simulink library "DQN_Lib (conflicted copy 2023-11-25 155310)"  (R2023b)
settings: Solver=VariableStepAuto  StartTime=0.0  StopTime=10.0  RelTol=1e-3
undefined symbols (not defined in the file): FreqRad, HrmOrd, Init, La, N, R, Ra, TimeStep, Ts, Ts_dqn, Ws
libraries: $bdroot x4, spsMeanVariableFrequencyLib x4, eeTransforms x3, spsabctodq0Lib x2, spsAlphaBetaZerotodq0Lib x1
(part 3 of 8)

== matlab function DQN_Lib (conflicted copy 2023-11-25 155310)/Mult_DQN_Mat ==
  data: X_DQN input; Y_DQN input; Z_DQN output; N parameter; HrmDbl parameter
function Z_DQN   = MultDQN(X_DQN, Y_DQN, N, HrmDbl)

    Xdp = X_DQN(:,1);
    Xdn = X_DQN(:,2);
    Xdz = X_DQN(:,3);
    Xqp = X_DQN(:,4);
    Xqn = X_DQN(:,5);
    Xqz = X_DQN(:,6);
    
    Ydp = Y_DQN(:,1);
    Ydn = Y_DQN(:,2);
    Ydz = Y_DQN(:,3);
    Yqp = Y_DQN(:,4);
    Yqn = Y_DQN(:,5);
    Yqz = Y_DQN(:,6);
    
    Z_DQN = zeros(2*N+1,6);

    Xdc = zeros(6,1);
    Ydc = zeros(6,1);
    Zdc = zeros(6,1);

    Xdc(1) = Xdp(1);
    Xdc(2) = Xdn(1);
    Xdc(3) = Xdz(1);
    Xdc(4) = Xqp(1);
    Xdc(5) = Xqn(1);
    Xdc(6) = Xqz(1);

    Ydc(1) = Ydp(1);
    Ydc(2) = Ydn(1);
    Ydc(3) = Ydz(1);
    Ydc(4) = Yqp(1);
    Ydc(5) = Yqn(1);
    Ydc(6) = Yqz(1);

    a = -0.5+0.866i;
    a2 = -0.5-0.866i;
    T = [1 1 1;1 a a2;1 a2 a];    

    Xdp = [Xdp(2:end); zeros(N-numel(Xdp)+1,1)];
    Ydp = [Ydp(2:end); zeros(N-numel(Ydp)+1,1)];
    Xqp = [Xqp(2:end); zeros(N-numel(Xqp)+1,1)];
    Yqp = [Yqp(2:end); zeros(N-numel(Yqp)+1,1)];
      
    Xdn = [Xdn(2:end); zeros(N-numel(Xdn)+1,1)];
    Ydn = [Ydn(2:end); zeros(N-numel(Ydn)+1,1)];
    Xqn = [Xqn(2:end); zeros(N-numel(Xqn)+1,1)];
    Yqn = [Yqn(2:end); zeros(N-numel(Yqn)+1,1)];
    
    Xdz = [Xdz(2:end); zeros(N-numel(Xdz)+1,1)];
    Ydz = [Ydz(2:end); zeros(N-numel(Ydz)+1,1)];
    Xqz = [Xqz(2:end); zeros(N-numel(Xqz)+1,1)];
    Yqz = [Yqz(2:end); zeros(N-numel(Yqz)+1,1)];
    
    Zdp = zeros(2*N+1,1);
    Zdn = zeros(2*N+1,1);
    Zdz = zeros(2*N+1,1);
    Zqp = zeros(2*N+1,1);
    Zqn = zeros(2*N+1,1);
    Zqz = zeros(2*N+1,1);
    
%    Tad_p =        [0  -0.577350269189626   0.577350269189626;
%    0.666666666666667  -0.333333333333333  -0.333333333333333;
%    0.333333333333333   0.333333333333333   0.333333333333333];

   Tad_p =        [0  -sqrt(3)/3   sqrt(3)/3;
                   2/3  -1/3  -1/3;
                   1/3   1/3   1/3];
    
%     Tad_p = (2/3)*[sin(0) sin(0-2*pi/3) sin(0+2*pi/3);  
%                    cos(0) cos(0-2*pi/3) cos(0+2*pi/3);
%                    0.5    0.5           0.5];

    Tda_p =  [-0           1     1;
              -sqrt(3)/2  -0.5   1;
               sqrt(3)/2  -0.5   1;];
    
    if(0)
    
       
    Zdc([1,4, 3]) = Tad_p*((Tda_p*Xdc([1,4,3])).*(Tda_p*Ydc([1,4,3])));
    
    else
        Tad_p = [0      -sqrt(1/3)   sqrt(1/3);
                (2/3)   -(1/3)      -(1/3);
                (1/3)    (1/3)       (1/3)];

        Tda_p = [-0           1     1;
                 -sqrt(3/4)  -0.5   1;
                  sqrt(3/4)  -0.5   1;];

    %     Tdqn_a = [Tda_p2(:,1)  Tda_p2(:,1)  Tda_z2(:,1)  Tda_p2(:,2)  Tda_p2(:,2)  2*Tda_z2(:,2)]/2;
    %     Ta_dqn = [Tad_p2(1,:); Tad_p2(1,:); Tad_z2(1,:); Tad_p2(2,:); Tad_p2(2,:); Tad_z2(2,:)];

        Tdqn_a = [Tda_p(:,1)  Tda_p(:,1)  0*Tda_p(:,3)  Tda_p(:,2)  Tda_p(:,2)  2*Tda_p(:,3)]/2;
        Ta_dqn = [Tad_p(1,:); Tad_p(1,:); 0*Tad_p(3,:); Tad_p(2,:); Tad_p(2,:); Tad_p(3,:)];
        

        Zdc = Ta_dqn*((Tdqn_a*Xdc).*(Tdqn_a*Ydc));


    end
    
         
    %Zdc = Xdc.*Ydc;
       
    for h = 1 : 2*N
        if(h<=N)

%             Zdc([1,4]) = Zdc([1,4]) + 0.5*(Xdp(h)*Ydp(h)+Xqp(h)*Yqp(h));
%             Zdc([2,5]) = Zdc([2,5]) + 0.5*(Xdn(h)*Ydn(h)+Xqn(h)*Yqn(h));
%             Zdc([3,6]) = Zdc([3,6]) + 0.5*(Xdz(h)*Ydz(h)+Xqz(h)*Yqz(h));
            
%             Zdc1 = Zdc1 + 0.5*(Xdp(h)*Ydp(h)+Xqp(h)*Yqp(h));
%             Zdc1 = Zdc1 + 0.5*(Xdn(h)*Ydn(h)+Xqn(h)*Yqn(h));
%             Zdc1 = Zdc1 + 0.5*(Xdz(h)*Ydz(h)+Xqz(h)*Yqz(h));
%             
            %Zdc([1,4, 3]) = Zdc([1,4, 3]) + Tad_p*0.5*(Xdp(h)*Ydp(h)+Xqp(h)*Yqp(h)+Xdn(h)*Ydn(h)+Xqn(h)*Yqn(h)+Xdz(h)*Ydz(h)+Xqz(h)*Yqz(h))*[1;1;1];
            Zdc = Zdc + Ta_dqn*0.5*((Xdp(h)*Ydp(h)+Xqp(h)*Yqp(h)+Xdn(h)*Ydn(h)+Xqn(h)*Yqn(h)+Xdz(h)*Ydz(h)+Xqz(h)*Yqz(h))*[1;1;1]);

            Ymp = sqrt(Ydp(h)^2+Yqp(h)^2);
            Yap = atan2(Yqp(h),+Ydp(h));  


            Ymn = sqrt(Ydn(h)^2+Yqn(h)^2);
            Yan = atan2(Yqn(h),-Ydn(h));  

            Xmz = sqrt(Xdz(h)^2+Xqz(h)^2);
            Xaz = atan2(Xqz(h),+Xdz(h));  
            Ymz = sqrt(Ydz(h)^2+Yqz(h)^2);
            Yaz = atan2(Yqz(h),+Ydz(h));  

            
            Xmp = sqrt(Xdp(h)^2+Xqp(h)^2);
            Xap = atan2(Xqp(h),+Xdp(h));  
            if(Xmp~=0)
            Zdz(2*h) = Zdz(2*h) + 0.5*Xmp*Ymn*sin(Xap+Yan);
            Zqz(2*h) = Zqz(2*h) - 0.5*Xmp*Ymn*cos(Xap+Yan);
%             Zdc([1,4,3]) = Zdc([1,4,3]) + Tad_p*0.5*Xmp*Ymn*[cos(Xap-Yan); cos(Xap-Yan-4*pi/3); cos(Xap-Yan+4*pi/3)];
%             Zdc([1,4,3]) = Zdc([1,4,3]) + Tad_p*0.5*Xmp*Ymz*[cos(Xap-Yaz); cos(Xap-Yaz+4*pi/3); cos(Xap-Yaz-4*pi/3)];
            Zdc = Zdc + Ta_dqn*0.5*Xmp*Ymn*[cos(Xap-Yan); cos(Xap-Yan-4*pi/3); cos(Xap-Yan+4*pi/3)];
            Zdc = Zdc + Ta_dqn*0.5*Xmp*Ymz*[cos(Xap-Yaz); cos(Xap-Yaz+4*pi/3); cos(Xap-Yaz-4*pi/3)];
            end

            Xmn = sqrt(Xdn(h)^2+Xqn(h)^2);
            Xan = atan2(Xqn(h),-Xdn(h));  
            if(Xmn~=0)
            Zdz(2*h) = Zdz(2*h) + 0.5*Xmn*Ymp*sin(Xan+Yap);
            Zqz(2*h) = Zqz(2*h) - 0.5*Xmn*Ymp*cos(Xan+Yap);
%             Zdc([1,4,3]) = Zdc([1,4,3]) + Tad_p*0.5*Xmn*Ymp*[cos(Xan-Yap); cos(Xan-Yap+4*pi/3); cos(Xan-Yap-4*pi/3)];
%             Zdc([1,4,3]) = Zdc([1,4,3]) + Tad_p*0.5*Xmn*Ymz*[cos(Xan-Yaz); cos(Xan-Yaz-4*pi/3); cos(Xan-Yaz+4*pi/3)];
            Zdc = Zdc + Ta_dqn*0.5*Xmn*Ymp*[cos(Xan-Yap); cos(Xan-Yap+4*pi/3); cos(Xan-Yap-4*pi/3)];
            Zdc = Zdc + Ta_dqn*0.5*Xmn*Ymz*[cos(Xan-Yaz); cos(Xan-Yaz-4*pi/3); cos(Xan-Yaz+4*pi/3)];
            end
            
            if(Xmz~=0)
%             Zdc([1,4,3]) = Zdc([1,4,3]) + Tad_p*0.5*Xmz*Ymp*[cos(Xaz-Yap); cos(Xaz-Yap-4*pi/3); cos(Xaz-Yap+4*pi/3)];
%             Zdc([1,4,3]) = Zdc([1,4,3]) + Tad_p*0.5*Xmz*Ymn*[cos(Xaz-Yan); cos(Xaz-Yan+4*pi/3); cos(Xaz-Yan-4*pi/3)];
            Zdc = Zdc + Ta_dqn*0.5*Xmz*Ymp*[cos(Xaz-Yap); cos(Xaz-Yap-4*pi/3); cos(Xaz-Yap+4*pi/3)];
            Zdc = Zdc + Ta_dqn*0.5*Xmz*Ymn*[cos(Xaz-Yan); cos(Xaz-Yan+4*pi/3); cos(Xaz-Yan-4*pi/3)];
            end

            if(all(Xdc == Xdc(1)) && all(Ydc == Ydc(1)))
                Zdp(h) = Zdp(h) + Xdc(1)*Ydp(h)+Xdp(h)*Ydc(1);     
                Zqp(h) = Zqp(h) + Xdc(1)*Yqp(h)+Xqp(h)*Ydc(1);  
                Zdn(h) = Zdn(h) + Xdc(1)*Ydn(h)+Xdn(h)*Ydc(1);
                Zqn(h) = Zqn(h) + Xdc(1)*Yqn(h)+Xqn(h)*Ydc(1);
                Zdz(h) = Zdz(h) + Xdc(1)*Ydz(h)+Xdz(h)*Ydc(1);     
                Zqz(h) = Zqz(h) + Xdc(1)*Yqz(h)+Xqz(h)*Ydc(1); 
            else
                %%%%%%%%%%%%%%%%% POSITIVE (Ydc*Xp) %%%%%%%%%%%%%%%%%%%
                if(Xmp ~= 0)
                    %Y_abc = Tda_p*Ydc([1,4,3]); 
                    Y_abc = Tdqn_a*Ydc; 
                    V_012 = T*[Y_abc(1)*Xmp*(cos(Xap)       +1i*sin(Xap));
                               Y_abc(2)*Xmp*(cos(Xap-2*pi/3)+1i*sin(Xap-2*pi/3));
                               Y_abc(3)*Xmp*(cos(Xap+2*pi/3)+1i*sin(Xap+2*pi/3))]/3;

                    Zdz(h) = Zdz(h) + real(V_012(1)); Zqz(h) = Zqz(h) + imag(V_012(1));
                    Zdp(h) = Zdp(h) + real(V_012(2)); Zqp(h) = Zqp(h) + imag(V_012(2));
                    Zdn(h) = Zdn(h) - real(V_012(3)); Zqn(h) = Zqn(h) + imag(V_012(3));
                end
                %%%%%%%%%%%%%%%%% POSITIVE (Xdc*Yp) %%%%%%%%%%%%%%%%%%%
                if(Ymp ~= 0)
                    %X_abc = Tda_p*Xdc([1,4,3]); 
                    X_abc = Tdqn_a*Xdc; 
                    V_012 = T*[X_abc(1)*Ymp*(cos(Yap)       +1i*sin(Yap));
                               X_abc(2)*Ymp*(cos(Yap-2*pi/3)+1i*sin(Yap-2*pi/3));
                               X_abc(3)*Ymp*(cos(Yap+2*pi/3)+1i*sin(Yap+2*pi/3))]/3;

                    Zdz(h) = Zdz(h) + real(V_012(1)); Zqz(h) = Zqz(h) + imag(V_012(1));
                    Zdp(h) = Zdp(h) + real(V_012(2)); Zqp(h) = Zqp(h) + imag(V_012(2));
                    Zdn(h) = Zdn(h) - real(V_012(3)); Zqn(h) = Zqn(h) + imag(V_012(3));
                end
                %%%%%%%%%%%%%%%%% NEGATIVE (Ydc*Xn) %%%%%%%%%%%%%%%%%%%
                if(Xmn ~= 0)
                    %Y_abc = Tda_p*Ydc([1,4,3]); 
                    Y_abc = Tdqn_a*Ydc; 
                    V_012 = T*[Y_abc(1)*Xmn*(cos(Xan)       +1i*sin(Xan));
                               Y_abc(2)*Xmn*(cos(Xan+2*pi/3)+1i*sin(Xan+2*pi/3));
                               Y_abc(3)*Xmn*(cos(Xan-2*pi/3)+1i*sin(Xan-2*pi/3))]/3;
                    

                    Zdz(h) = Zdz(h) + real(V_012(1)); Zqz(h) = Zqz(h) + imag(V_012(1));
                    Zdp(h) = Zdp(h) + real(V_012(2)); Zqp(h) = Zqp(h) + imag(V_012(2));
                    Zdn(h) = Zdn(h) - real(V_012(3)); Zqn(h) = Zqn(h) + imag(V_012(3));
                end
                %%%%%%%%%%%%%%%%% NEGATIVE (Xdc*Yn) %%%%%%%%%%%%%%%%%%%
                if(Ymn ~= 0)
                    %X_abc = Tda_p*Xdc([1,4,3]); 
                    X_abc = Tdqn_a*Xdc; 
                    V_012 = T*[X_abc(1)*Ymn*(cos(Yan)       +1i*sin(Yan));
                               X_abc(2)*Ymn*(cos(Yan+2*pi/3)+1i*sin(Yan+2*pi/3));
                               X_abc(3)*Ymn*(cos(Yan-2*pi/3)+1i*sin(Yan-2*pi/3))]/3;

                    Zdz(h) = Zdz(h) + real(V_012(1)); Zqz(h) = Zqz(h) + imag(V_012(1));
                    Zdp(h) = Zdp(h) + real(V_012(2)); Zqp(h) = Zqp(h) + imag(V_012(2));
                    Zdn(h) = Zdn(h) - real(V_012(3)); Zqn(h) = Zqn(h) + imag(V_012(3));
                end
                %%%%%%%%%%%%%%%%%%%%%%%%%%%%%%%%%%%%%%%%%%%%%%%%%%%%%%
                if(Xmz ~= 0)
                    %Y_abc = Tda_p*Ydc([1,4,3]); 
                    Y_abc = Tdqn_a*Ydc; 
                    V_012 = T*[Y_abc(1)*Xmz*(cos(Xaz)+1i*sin(Xaz));
                               Y_abc(2)*Xmz*(cos(Xaz)+1i*sin(Xaz));
                               Y_abc(3)*Xmz*(cos(Xaz)+1i*sin(Xaz))]/3;
                    
                    Zdz(h) = Zdz(h) + real(V_012(1)); Zqz(h) = Zqz(h) + imag(V_012(1));
                    Zdp(h) = Zdp(h) + real(V_012(2)); Zqp(h) = Zqp(h) + imag(V_012(2));
                    Zdn(h) = Zdn(h) - real(V_012(3)); Zqn(h) = Zqn(h) + imag(V_012(3));
                end
                %%%%%%%%%%%%%%%%%%%%%%%%%%%%%%%%%%%%%%%%%%%%%%%%%%%%%%

                if(Ymz ~= 0)
                    %X_abc = Tda_p*Xdc([1,4,3]); 
                    X_abc = Tdqn_a*Xdc; 
                    V_012 = T*[X_abc(1)*Ymz*(cos(Yaz)+1i*sin(Yaz));
                               X_abc(2)*Ymz*(cos(Yaz)+1i*sin(Yaz));
                               X_abc(3)*Ymz*(cos(Yaz)+1i*sin(Yaz))]/3;
                    
                    Zdz(h) = Zdz(h) + real(V_012(1)); Zqz(h) = Zqz(h) + imag(V_012(1));
                    Zdp(h) = Zdp(h) + real(V_012(2)); Zqp(h) = Zqp(h) + imag(V_012(2));
                    Zdn(h) = Zdn(h) - real(V_012(3)); Zqn(h) = Zqn(h) + imag(V_012(3));
                end
            end
            
%%%%%%%%%%%%%%%%%%%%%% h<=N ODD %%%%%%%%%%%%%%%%%%%%%%%%%%%%%%%%%%%%%%%%%
            if(mod(h,2)==1) 
                %%%%%%%%%%%%%%%%% D3p (3ph+) %%%%%%%%%%%%%%%%%%%%%%%

                %&%%%%%%%%%%%%%%%%%%%%%%%%%% PP + NN %%%%%%%%%%%%%%%%%%%%%%%%%%%
                for i = 1 : h - 1
                   Zdp(h) = Zdp(h) - 0.5*(Xdn(i)*Yqn(h-i) + Xqn(i)*Ydn(h-i));                    
                   Zdn(h) = Zdn(h) - 0.5*(Xdp(i)*Yqp(h-i) + Xqp(i)*Ydp(h-i)); 
                   Zqp(h) = Zqp(h) - 0.5*(Xdn(i)*Ydn(h-i) - Xqn(i)*Yqn(h-i));                
                   Zqn(h) = Zqn(h) - 0.5*(Xdp(i)*Ydp(h-i) - Xqp(i)*Yqp(h-i)); 
                end

                for i = 1 : N - h
                    Zdz(h) = Zdz(h) + 0.5*(-Xdp(i)*Yqp(i+h) + Xqp(i)*Ydp(i+h) + Xdp(i+h)*Yqp(i) - Xqp(i+h)*Ydp(i) + Xdn(i)*Yqn(i+h) - Xqn(i)*Ydn(i+h) - Xdn(i+h)*Yqn(i) + Xqn(i+h)*Ydn(i));  
                    Zqz(h) = Zqz(h) + 0.5*(+Xdp(i)*Ydp(i+h) + Xqp(i)*Yqp(i+h) + Xdp(i+h)*Ydp(i) + Xqp(i+h)*Yqp(i) + Xdn(i)*Ydn(i+h) + Xqn(i)*Yqn(i+h) + Xdn(i+h)*Ydn(i) + Xqn(i+h)*Yqn(i));    
                end
                %&%%%%%%%%%%%%%%%%%%%%%%%%%% PP + NN %%%%%%%%%%%%%%%%%%%%%%%%%%%

                for k = 1 : (N + mod(N+1,2) - h)/2
                    i = 2*k-1;
                    j = i+h;

                    Zdz(h)  = Zdz(h)  + 0.5*(-Xdz(i)*Yqz(j) + Xqz(i)*Ydz(j) + Xdz(j)*Yqz(i) - Xqz(j)*Ydz(i));
                    Zqz(h)  = Zqz(h)  + 0.5*(+Xdz(i)*Ydz(j) + Xqz(i)*Yqz(j) + Xdz(j)*Ydz(i) + Xqz(j)*Yqz(i)); 

                    Zdp(h) = Zdp(h) + 0.5*(-Xdp(i)*Yqn(j) - Xqp(i)*Ydn(j) - Xdn(j)*Yqp(i) - Xqn(j)*Ydp(i)); 
                    Zdp(h) = Zdp(h) + 0.5*(-Xdz(i)*Yqp(j) + Xqz(i)*Ydp(j) + Xdp(j)*Yqz(i) - Xqp(j)*Ydz(i));    
                    Zdp(h) = Zdp(h) + 0.5*(+Xdn(i)*Yqz(j) + Xqn(i)*Ydz(j) + Xdz(j)*Yqn(i) + Xqz(j)*Ydn(i));
                    
                    Zqp(h) = Zqp(h) + 0.5*(-Xdp(i)*Ydn(j) + Xqp(i)*Yqn(j) - Xdn(j)*Ydp(i) + Xqn(j)*Yqp(i));  
                    Zqp(h) = Zqp(h) + 0.5*(+Xdz(i)*Ydp(j) + Xqz(i)*Yqp(j) + Xdp(j)*Ydz(i) + Xqp(j)*Yqz(i));     
                    Zqp(h) = Zqp(h) + 0.5*(-Xdn(i)*Ydz(j) + Xqn(i)*Yqz(j) - Xdz(j)*Ydn(i) + Xqz(j)*Yqn(i));

                    Zdn(h) = Zdn(h) + 0.5*(+Xdp(i)*Yqz(j) - Xqp(i)*Ydz(j) - Xdz(j)*Yqp(i) + Xqz(j)*Ydp(i));             
                    Zdn(h) = Zdn(h) + 0.5*(+Xdz(i)*Yqn(j) + Xqz(i)*Ydn(j) + Xdn(j)*Yqz(i) + Xqn(j)*Ydz(i));
                    Zdn(h) = Zdn(h) + 0.5*(-Xdn(i)*Yqp(j) - Xqn(i)*Ydp(j) - Xdp(j)*Yqn(i) - Xqp(j)*Ydn(i)); 

                    Zqn(h) = Zqn(h) + 0.5*(+Xdp(i)*Ydz(j) + Xqp(i)*Yqz(j) + Xdz(j)*Ydp(i) + Xqz(j)*Yqp(i)); 
                    Zqn(h) = Zqn(h) + 0.5*(-Xdz(i)*Ydn(j) + Xqz(i)*Yqn(j) - Xdn(j)*Ydz(i) + Xqn(j)*Yqz(i)); 
                    Zqn(h) = Zqn(h) + 0.5*(-Xdn(i)*Ydp(j) + Xqn(i)*Yqp(j) - Xdp(j)*Ydn(i) + Xqp(j)*Yqn(i));  
                end

                for k = 1 : (N + mod(N,2) - h - 1)/2
                    i = 2*k;
                    j = i+h;
                    
                    Zdz(h) = Zdz(h)   + 0.5*(-Xdz(i)*Yqz(j) + Xqz(i)*Ydz(j) + Xdz(j)*Yqz(i) - Xqz(j)*Ydz(i));
                    Zqz(h) = Zqz(h)   + 0.5*(+Xdz(i)*Ydz(j) + Xqz(i)*Yqz(j) + Xdz(j)*Ydz(i) + Xqz(j)*Yqz(i)); 

                    Zdp(h) = Zdp(h) + 0.5*(-Xdp(i)*Yqn(j) - Xqp(i)*Ydn(j) - Xdn(j)*Yqp(i) - Xqn(j)*Ydp(i)); 
                    Zqp(h) = Zqp(h) + 0.5*(-Xdp(i)*Ydn(j) + Xqp(i)*Yqn(j) - Xdn(j)*Ydp(i) + Xqn(j)*Yqp(i));  
                    Zdn(h) = Zdn(h) + 0.5*(-Xdn(i)*Yqp(j) - Xqn(i)*Ydp(j) - Xdp(j)*Yqn(i) - Xqp(j)*Ydn(i)); 
                    Zqn(h) = Zqn(h) + 0.5*(-Xdn(i)*Ydp(j) + Xqn(i)*Yqp(j) - Xdp(j)*Ydn(i) + Xqp(j)*Yqn(i));                                          

                    Zdp(h) = Zdp(h) + 0.5*(-Xdz(i)*Yqp(j) + Xqz(i)*Ydp(j) + Xdp(j)*Yqz(i) - Xqp(j)*Ydz(i));
                    Zqp(h) = Zqp(h) + 0.5*(+Xdz(i)*Ydp(j) + Xqz(i)*Yqp(j) + Xdp(j)*Ydz(i) + Xqp(j)*Yqz(i));                     
                    Zdn(h) = Zdn(h) + 0.5*(+Xdp(i)*Yqz(j) - Xqp(i)*Ydz(j) - Xdz(j)*Yqp(i) + Xqz(j)*Ydp(i));
                    Zqn(h) = Zqn(h) + 0.5*(+Xdp(i)*Ydz(j) + Xqp(i)*Yqz(j) + Xdz(j)*Ydp(i) + Xqz(j)*Yqp(i));   

                    Zdp(h) = Zdp(h) + 0.5*(+Xdn(i)*Yqz(j) + Xqn(i)*Ydz(j) + Xdz(j)*Yqn(i) + Xqz(j)*Ydn(i));
                    Zqp(h) = Zqp(h) + 0.5*(-Xdn(i)*Ydz(j) + Xqn(i)*Yqz(j) - Xdz(j)*Ydn(i) + Xqz(j)*Yqn(i));                
                    Zdn(h) = Zdn(h) + 0.5*(+Xdz(i)*Yqn(j) + Xqz(i)*Ydn(j) + Xdn(j)*Yqz(i) + Xqn(j)*Ydz(i));
                    Zqn(h) = Zqn(h) + 0.5*(-Xdz(i)*Ydn(j) + Xqz(i)*Yqn(j) - Xdn(j)*Ydz(i) + Xqn(j)*Yqz(i)); 

                end

                for k = (h-1)/2:-1:1
                    i = k;
                    j = h-i;  
                    
                    Zdz(h) = Zdz(h) + 0.5*(+Xdp(i)*Yqn(j)-Xqp(i)*Ydn(j)-Xdn(j)*Yqp(i)+Xqn(j)*Ydp(i));
                    Zqz(h) = Zqz(h) + 0.5*(+Xdp(i)*Ydn(j)+Xqp(i)*Yqn(j)+Xdn(j)*Ydp(i)+Xqn(j)*Yqp(i));
                    Zdz(h) = Zdz(h) + 0.5*(+Xdp(j)*Yqn(i)-Xqp(j)*Ydn(i)-Xdn(i)*Yqp(j)+Xqn(i)*Ydp(j));
                    Zqz(h) = Zqz(h) + 0.5*(+Xdp(j)*Ydn(i)+Xqp(j)*Yqn(i)+Xdn(i)*Ydp(j)+Xqn(i)*Yqp(j)); 
                    Zdz(h) = Zdz(h) + 0.5*(+Xdz(i)*Yqz(j)+Xqz(i)*Ydz(j)+Xdz(j)*Yqz(i)+Xqz(j)*Ydz(i));
                    Zqz(h) = Zqz(h) + 0.5*(-Xdz(i)*Ydz(j)+Xqz(i)*Yqz(j)-Xdz(j)*Ydz(i)+Xqz(j)*Yqz(i));    
                        
                        
                    Zdp(h) = Zdp(h) + 0.5*(+Xdz(i)*Yqp(j)+Xqz(i)*Ydp(j)+Xdz(j)*Yqp(i)+Xqz(j)*Ydp(i));
                    Zqp(h) = Zqp(h) + 0.5*(-Xdz(i)*Ydp(j)+Xqz(i)*Yqp(j)-Xdz(j)*Ydp(i)+Xqz(j)*Yqp(i));
                    Zdp(h) = Zdp(h) + 0.5*(+Xdp(i)*Yqz(j)+Xqp(i)*Ydz(j)+Xdp(j)*Yqz(i)+Xqp(j)*Ydz(i));
                    Zqp(h) = Zqp(h) + 0.5*(-Xdp(i)*Ydz(j)+Xqp(i)*Yqz(j)-Xdp(j)*Ydz(i)+Xqp(j)*Yqz(i)); 
                    
                              
                    Zdn(h) = Zdn(h) + 0.5*(+Xdn(i)*Yqz(j)-Xqn(i)*Ydz(j)+Xdn(j)*Yqz(i)-Xqn(j)*Ydz(i));
                    Zqn(h) = Zqn(h) + 0.5*(+Xdn(i)*Ydz(j)+Xqn(i)*Yqz(j)+Xdn(j)*Ydz(i)+Xqn(j)*Yqz(i)); 
                    Zdn(h) = Zdn(h) + 0.5*(-Xdz(i)*Yqn(j)+Xqz(i)*Ydn(j)-Xdz(j)*Yqn(i)+Xqz(j)*Ydn(i));
                    Zqn(h) = Zqn(h) + 0.5*(+Xdz(i)*Ydn(j)+Xqz(i)*Yqn(j)+Xdz(j)*Ydn(i)+Xqz(j)*Yqn(i)); 
                end
%%%%%%%%%%%%%%%%%%%%%% h<=N EVEN %%%%%%%%%%%%%%%%%%%%%%%%%%%%%%%%%%%%%%%%%           
            else 
               
                Zdp(h) = Zdp(h) + 0.5*(-Xdn(h/2)*Yqn(h/2)-Xqn(h/2)*Ydn(h/2));   
                Zqp(h) = Zqp(h) + 0.5*(-Xdn(h/2)*Ydn(h/2)+Xqn(h/2)*Yqn(h/2)); 
                Zdn(h) = Zdn(h) + 0.5*(-Xdp(h/2)*Yqp(h/2)-Xqp(h/2)*Ydp(h/2));   
                Zqn(h) = Zqn(h) + 0.5*(-Xdp(h/2)*Ydp(h/2)+Xqp(h/2)*Yqp(h/2));   

                Zdz(h)  = Zdz(h)  + 0.5*(+Xdz(h/2)*Yqz(h/2)+Xqz(h/2)*Ydz(h/2));
                Zqz(h)  = Zqz(h)  + 0.5*(-Xdz(h/2)*Ydz(h/2)+Xqz(h/2)*Yqz(h/2));

                Zdp(h) = Zdp(h) + 0.5*(+Xdz(h/2)*Yqp(h/2)+Xqz(h/2)*Ydp(h/2)+Xdp(h/2)*Yqz(h/2)+Xqp(h/2)*Ydz(h/2));   
                Zqp(h) = Zqp(h) + 0.5*(-Xdz(h/2)*Ydp(h/2)+Xqz(h/2)*Yqp(h/2)-Xdp(h/2)*Ydz(h/2)+Xqp(h/2)*Yqz(h/2)); 
                Zdn(h) = Zdn(h) + 0.5*(+Xdn(h/2)*Yqz(h/2)-Xqn(h/2)*Ydz(h/2)-Xdz(h/2)*Yqn(h/2)+Xqz(h/2)*Ydn(h/2));   
                Zqn(h) = Zqn(h) + 0.5*(+Xdn(h/2)*Ydz(h/2)+Xqn(h/2)*Yqz(h/2)+Xdz(h/2)*Ydn(h/2)+Xqz(h/2)*Yqn(h/2));    
                
                for k = 1:N-h
                    i = k;
                    j = h+i;
                
                    Zdz(h) = Zdz(h)   + 0.5*(+Xdp(j)*Yqp(i) - Xqp(j)*Ydp(i) - Xdp(i)*Yqp(j) + Xqp(i)*Ydp(j));
                    Zqz(h) = Zqz(h)   + 0.5*(+Xdp(j)*Ydp(i) + Xqp(j)*Yqp(i) + Xdp(i)*Ydp(j) + Xqp(i)*Yqp(j));                                           
                    Zdz(h) = Zdz(h)   + 0.5*(+Xdn(i)*Yqn(j) - Xqn(i)*Ydn(j) - Xdn(j)*Yqn(i) + Xqn(j)*Ydn(i));
                    Zqz(h) = Zqz(h)   + 0.5*(+Xdn(i)*Ydn(j) + Xqn(i)*Yqn(j) + Xdn(j)*Ydn(i) + Xqn(j)*Yqn(i));  
                    Zdz(h) = Zdz(h)   + 0.5*(-Xdz(i)*Yqz(j) + Xqz(i)*Ydz(j) + Xdz(j)*Yqz(i) - Xqz(j)*Ydz(i));
                    Zqz(h) = Zqz(h)   + 0.5*(+Xdz(i)*Ydz(j) + Xqz(i)*Yqz(j) + Xdz(j)*Ydz(i) + Xqz(j)*Yqz(i)); 
                                       
                    Zdp(h) = Zdp(h) + 0.5*(-Xdp(i)*Yqn(j) - Xqp(i)*Ydn(j) - Xdn(j)*Yqp(i) - Xqn(j)*Ydp(i)); 
                    Zqp(h) = Zqp(h) + 0.5*(-Xdp(i)*Ydn(j) + Xqp(i)*Yqn(j) - Xdn(j)*Ydp(i) + Xqn(j)*Yqp(i)); 
                    Zdn(h) = Zdn(h) + 0.5*(-Xdn(i)*Yqp(j) - Xqn(i)*Ydp(j) - Xdp(j)*Yqn(i) - Xqp(j)*Ydn(i)); 
                    Zqn(h) = Zqn(h) + 0.5*(-Xdn(i)*Ydp(j) + Xqn(i)*Yqp(j) - Xdp(j)*Ydn(i) + Xqp(j)*Yqn(i)); 
                        
                    Zdp(h) = Zdp(h) + 0.5*(+Xdp(j)*Yqz(i) - Xqp(j)*Ydz(i) - Xdz(i)*Yqp(j) + Xqz(i)*Ydp(j));
                    Zqp(h) = Zqp(h) + 0.5*(+Xdp(j)*Ydz(i) + Xqp(j)*Yqz(i) + Xdz(i)*Ydp(j) + Xqz(i)*Yqp(j)); 
                    Zdn(h) = Zdn(h) + 0.5*(+Xdp(i)*Yqz(j) - Xqp(i)*Ydz(j) - Xdz(j)*Yqp(i) + Xqz(j)*Ydp(i));
                    Zqn(h) = Zqn(h) + 0.5*(+Xdp(i)*Ydz(j) + Xqp(i)*Yqz(j) + Xdz(j)*Ydp(i) + Xqz(j)*Yqp(i)); 
                    
                    Zdp(h) = Zdp(h) + 0.5*(+Xdn(i)*Yqz(j) + Xqn(i)*Ydz(j) + Xdz(j)*Yqn(i) + Xqz(j)*Ydn(i));
                    Zqp(h) = Zqp(h) + 0.5*(-Xdn(i)*Ydz(j) + Xqn(i)*Yqz(j) - Xdz(j)*Ydn(i) + Xqz(j)*Yqn(i)); 
                    Zdn(h) = Zdn(h) + 0.5*(+Xdn(j)*Yqz(i) + Xqn(j)*Ydz(i) + Xdz(i)*Yqn(j) + Xqz(i)*Ydn(j));
                    Zqn(h) = Zqn(h) + 0.5*(-Xdn(j)*Ydz(i) + Xqn(j)*Yqz(i) - Xdz(i)*Ydn(j) + Xqz(i)*Yqn(j)); 
                end

                for k = h/2-1:-1:1
                    i = k;
                    j = h-i;   

                    Zdz(h) = Zdz(h)   + 0.5*(+Xdp(i)*Yqn(j) - Xqp(i)*Ydn(j) + Xdp(j)*Yqn(i) - Xqp(j)*Ydn(i));
                    Zdz(h) = Zdz(h)   + 0.5*(-Xdn(i)*Yqp(j) + Xqn(i)*Ydp(j) - Xdn(j)*Yqp(i) + Xqn(j)*Ydp(i));      
                    Zdz(h) = Zdz(h)   + 0.5*(+Xdz(i)*Yqz(j) + Xqz(i)*Ydz(j) + Xdz(j)*Yqz(i) + Xqz(j)*Ydz(i));
                    
                    Zqz(h) = Zqz(h)   + 0.5*(+Xdp(i)*Ydn(j) + Xqp(i)*Yqn(j) + Xdp(j)*Ydn(i) + Xqp(j)*Yqn(i)); 
                    Zqz(h) = Zqz(h)   + 0.5*(+Xdn(i)*Ydp(j) + Xqn(i)*Yqp(j) + Xdn(j)*Ydp(i) + Xqn(j)*Yqp(i));
                    Zqz(h) = Zqz(h)   + 0.5*(-Xdz(i)*Ydz(j) + Xqz(i)*Yqz(j) - Xdz(j)*Ydz(i) + Xqz(j)*Yqz(i)); 
                    
                    Zdp(h) = Zdp(h) + 0.5*(+Xdp(i)*Yqz(j) + Xqp(i)*Ydz(j) + Xdp(j)*Yqz(i) + Xqp(j)*Ydz(i)); 
                    Zdp(h) = Zdp(h) + 0.5*(-Xdn(i)*Yqn(j) - Xqn(i)*Ydn(j) - Xdn(j)*Yqn(i) - Xqn(j)*Ydn(i)); 
                    Zdp(h) = Zdp(h) + 0.5*(+Xdz(i)*Yqp(j) + Xqz(i)*Ydp(j) + Xdz(j)*Yqp(i) + Xqz(j)*Ydp(i));
                    
                    Zqp(h) = Zqp(h) + 0.5*(-Xdp(i)*Ydz(j) + Xqp(i)*Yqz(j) - Xdp(j)*Ydz(i) + Xqp(j)*Yqz(i)); 
                    Zqp(h) = Zqp(h) + 0.5*(-Xdn(i)*Ydn(j) + Xqn(i)*Yqn(j) - Xdn(j)*Ydn(i) + Xqn(j)*Yqn(i));
                    Zqp(h) = Zqp(h) + 0.5*(-Xdz(i)*Ydp(j) + Xqz(i)*Yqp(j) - Xdz(j)*Ydp(i) + Xqz(j)*Yqp(i));  
                    
                    Zdn(h) = Zdn(h) + 0.5*(-Xdp(i)*Yqp(j) - Xqp(i)*Ydp(j) - Xdp(j)*Yqp(i) - Xqp(j)*Ydp(i));
                    Zdn(h) = Zdn(h) + 0.5*(+Xdn(i)*Yqz(j) - Xqn(i)*Ydz(j) + Xdn(j)*Yqz(i) - Xqn(j)*Ydz(i));
                    Zdn(h) = Zdn(h) + 0.5*(-Xdz(i)*Yqn(j) + Xqz(i)*Ydn(j) - Xdz(j)*Yqn(i) + Xqz(j)*Ydn(i));
                    
                    Zqn(h) = Zqn(h) + 0.5*(-Xdp(i)*Ydp(j) + Xqp(i)*Yqp(j) - Xdp(j)*Ydp(i) + Xqp(j)*Yqp(i));  
                    Zqn(h) = Zqn(h) + 0.5*(+Xdn(i)*Ydz(j) + Xqn(i)*Yqz(j) + Xdn(j)*Ydz(i) + Xqn(j)*Yqz(i));
                    Zqn(h) = Zqn(h) + 0.5*(+Xdz(i)*Ydn(j) + Xqz(i)*Yqn(j) + Xdz(j)*Ydn(i) + Xqz(j)*Yqn(i)); 
                end
            end
%%%%%%%%%%%%%%%%%%%%%%%%%%%% h>N  %%%%%%%%%%%%%%%%%%%%%%%%%%%%%%%%%%%%%%%%% 
        else %h>N
            if(HrmDbl)
            
                %%%%%%%%%%%%%%%%%%%%%%%%%%% PP + NN %%%%%%%%%%%%%%%%%%%%%%%%%%%
                for i = h-N : N
                    Zdp(h) = Zdp(h) - 0.5*(Xdn(i)*Yqn(h-i) + Xqn(i)*Ydn(h-i));                
                    Zdn(h) = Zdn(h) - 0.5*(Xdp(i)*Yqp(h-i) + Xqp(i)*Ydp(h-i));                     
                    Zqp(h) = Zqp(h) - 0.5*(Xdn(i)*Ydn(h-i) - Xqn(i)*Yqn(h-i));                      
                    Zqn(h) = Zqn(h) - 0.5*(Xdp(i)*Ydp(h-i) - Xqp(i)*Yqp(h-i));   
                end
                %%%%%%%%%%%%%%%%%%%%%%%%%%% PP + NN %%%%%%%%%%%%%%%%%%%%%%%%%%%

                if(mod(h,2)==1) %%%%%%%%%%% h>N ODD %%%%%%%%%%%%%%%%%%%

                    for k = (h-1)/2:-1:h-N
                        i = k;
                        j = h-i;

                        Zdz(h) = Zdz(h) + 0.5*(+Xdp(i)*Yqn(j)-Xqp(i)*Ydn(j)-Xdn(j)*Yqp(i)+Xqn(j)*Ydp(i));                  
                        Zdz(h) = Zdz(h) + 0.5*(+Xdp(j)*Yqn(i)-Xqp(j)*Ydn(i)-Xdn(i)*Yqp(j)+Xqn(i)*Ydp(j));
                        Zdz(h) = Zdz(h) + 0.5*(+Xdz(i)*Yqz(j)+Xqz(i)*Ydz(j)+Xdz(j)*Yqz(i)+Xqz(j)*Ydz(i));

                        Zqz(h) = Zqz(h) + 0.5*(-Xdz(i)*Ydz(j)+Xqz(i)*Yqz(j)-Xdz(j)*Ydz(i)+Xqz(j)*Yqz(i));
                        Zqz(h) = Zqz(h) + 0.5*(+Xdp(i)*Ydn(j)+Xqp(i)*Yqn(j)+Xdn(j)*Ydp(i)+Xqn(j)*Yqp(i));
                        Zqz(h) = Zqz(h) + 0.5*(+Xdp(j)*Ydn(i)+Xqp(j)*Yqn(i)+Xdn(i)*Ydp(j)+Xqn(i)*Yqp(j));  

                        Zdp(h) = Zdp(h) + 0.5*(+Xdp(i)*Yqz(j)+Xqp(i)*Ydz(j)+Xdp(j)*Yqz(i)+Xqp(j)*Ydz(i));
                        Zdp(h) = Zdp(h) + 0.5*(+Xdz(i)*Yqp(j)+Xqz(i)*Ydp(j)+Xdz(j)*Yqp(i)+Xqz(j)*Ydp(i));

                        Zqp(h) = Zqp(h) + 0.5*(-Xdp(i)*Ydz(j)+Xqp(i)*Yqz(j)-Xdp(j)*Ydz(i)+Xqp(j)*Yqz(i)); 
                        Zqp(h) = Zqp(h) + 0.5*(-Xdz(i)*Ydp(j)+Xqz(i)*Yqp(j)-Xdz(j)*Ydp(i)+Xqz(j)*Yqp(i));     

                        Zdn(h) = Zdn(h) + 0.5*(+Xdn(i)*Yqz(j)-Xqn(i)*Ydz(j)+Xdn(j)*Yqz(i)-Xqn(j)*Ydz(i));
                        Zdn(h) = Zdn(h) + 0.5*(-Xdz(i)*Yqn(j)+Xqz(i)*Ydn(j)-Xdz(j)*Yqn(i)+Xqz(j)*Ydn(i));

                        Zqn(h) = Zqn(h) + 0.5*(+Xdn(i)*Ydz(j)+Xqn(i)*Yqz(j)+Xdn(j)*Ydz(i)+Xqn(j)*Yqz(i));
                        Zqn(h) = Zqn(h) + 0.5*(+Xdz(i)*Ydn(j)+Xqz(i)*Yqn(j)+Xdz(j)*Ydn(i)+Xqz(j)*Yqn(i));    

                    end

                else %%%%%%%%%%% h>N EVEN %%%%%%%%%%%%%%%%%%%

                    Zdz(h)  = Zdz(h)  + 0.5*(+Xdz(h/2)*Yqz(h/2)+Xqz(h/2)*Ydz(h/2));
                    Zqz(h)  = Zqz(h)  + 0.5*(-Xdz(h/2)*Ydz(h/2)+Xqz(h/2)*Yqz(h/2));

                    Zdp(h) = 0.5*(-Xdn(h/2)*Yqn(h/2)-Xqn(h/2)*Ydn(h/2));          
                    Zdp(h) = Zdp(h) + 0.5*(+Xdp(h/2)*Yqz(h/2)+Xqp(h/2)*Ydz(h/2));                
                    Zdp(h) = Zdp(h) + 0.5*(+Xdz(h/2)*Yqp(h/2)+Xqz(h/2)*Ydp(h/2));    

                    Zqp(h) = 0.5*(-Xdn(h/2)*Ydn(h/2)+Xqn(h/2)*Yqn(h/2));             
                    Zqp(h) = Zqp(h) + 0.5*(-Xdp(h/2)*Ydz(h/2)+Xqp(h/2)*Yqz(h/2));        
                    Zqp(h) = Zqp(h) + 0.5*(-Xdz(h/2)*Ydp(h/2)+Xqz(h/2)*Yqp(h/2)); 

                    Zdn(h) = 0.5*(-Xdp(h/2)*Yqp(h/2)-Xqp(h/2)*Ydp(h/2)); 
                    Zdn(h) = Zdn(h) + 0.5*(+Xdn(h/2)*Yqz(h/2)-Xqn(h/2)*Ydz(h/2));
                    Zdn(h) = Zdn(h) + 0.5*(-Xdz(h/2)*Yqn(h/2)+Xqz(h/2)*Ydn(h/2));

                    Zqn(h) = 0.5*(-Xdp(h/2)*Ydp(h/2)+Xqp(h/2)*Yqp(h/2)); 
                    Zqn(h) = Zqn(h) + 0.5*(+Xdn(h/2)*Ydz(h/2)+Xqn(h/2)*Yqz(h/2));        
                    Zqn(h) = Zqn(h) + 0.5*(+Xdz(h/2)*Ydn(h/2)+Xqz(h/2)*Yqn(h/2)); 

                    for i = (h+2)/2:N
                        j = h-i;
                        Zdz(h)  = Zdz(h)  + 0.5*(+Xdp(i)*Yqn(j)-Xqp(i)*Ydn(j)+Xdp(j)*Yqn(i)-Xqp(j)*Ydn(i));
                        Zdz(h)  = Zdz(h)  + 0.5*(-Xdn(i)*Yqp(j)+Xqn(i)*Ydp(j)-Xdn(j)*Yqp(i)+Xqn(j)*Ydp(i));
                        Zdz(h)  = Zdz(h)  + 0.5*(+Xdz(i)*Yqz(j)+Xqz(i)*Ydz(j)+Xdz(j)*Yqz(i)+Xqz(j)*Ydz(i));

                        Zqz(h)  = Zqz(h)  + 0.5*(+Xdp(i)*Ydn(j)+Xqp(i)*Yqn(j)+Xdp(j)*Ydn(i)+Xqp(j)*Yqn(i));                      
                        Zqz(h)  = Zqz(h)  + 0.5*(+Xdn(i)*Ydp(j)+Xqn(i)*Yqp(j)+Xdn(j)*Ydp(i)+Xqn(j)*Yqp(i));  
                        Zqz(h)  = Zqz(h)  + 0.5*(-Xdz(i)*Ydz(j)+Xqz(i)*Yqz(j)-Xdz(j)*Ydz(i)+Xqz(j)*Yqz(i));

                        Zdp(h) = Zdp(h) + 0.5*(+Xdp(i)*Yqz(j)+Xqp(i)*Ydz(j)+Xdp(j)*Yqz(i)+Xqp(j)*Ydz(i));  
                        Zdp(h) = Zdp(h) + 0.5*(-Xdn(i)*Yqn(j)-Xqn(i)*Ydn(j)-Xdn(j)*Yqn(i)-Xqn(j)*Ydn(i));             
                        Zdp(h) = Zdp(h) + 0.5*(+Xdz(i)*Yqp(j)+Xqz(i)*Ydp(j)+Xdz(j)*Yqp(i)+Xqz(j)*Ydp(i));           

                        Zqp(h) = Zqp(h) + 0.5*(-Xdp(i)*Ydz(j)+Xqp(i)*Yqz(j)-Xdp(j)*Ydz(i)+Xqp(j)*Yqz(i));
                        Zqp(h) = Zqp(h) + 0.5*(-Xdn(i)*Ydn(j)+Xqn(i)*Yqn(j)-Xdn(j)*Ydn(i)+Xqn(j)*Yqn(i));    
                        Zqp(h) = Zqp(h) + 0.5*(-Xdz(i)*Ydp(j)+Xqz(i)*Yqp(j)-Xdz(j)*Ydp(i)+Xqz(j)*Yqp(i));   

                        Zdn(h) = Zdn(h) + 0.5*(-Xdp(i)*Yqp(j)-Xqp(i)*Ydp(j)-Xdp(j)*Yqp(i)-Xqp(j)*Ydp(i));
                        Zdn(h) = Zdn(h) + 0.5*(+Xdn(i)*Yqz(j)-Xqn(i)*Ydz(j)+Xdn(j)*Yqz(i)-Xqn(j)*Ydz(i));
                        Zdn(h) = Zdn(h) + 0.5*(-Xdz(i)*Yqn(j)+Xqz(i)*Ydn(j)-Xdz(j)*Yqn(i)+Xqz(j)*Ydn(i));              

                        Zqn(h) = Zqn(h) + 0.5*(-Xdp(i)*Ydp(j)+Xqp(i)*Yqp(j)-Xdp(j)*Ydp(i)+Xqp(j)*Yqp(i));
                        Zqn(h) = Zqn(h) + 0.5*(+Xdn(i)*Ydz(j)+Xqn(i)*Yqz(j)+Xdn(j)*Ydz(i)+Xqn(j)*Yqz(i)); 
                        Zqn(h) = Zqn(h) + 0.5*(+Xdz(i)*Ydn(j)+Xqz(i)*Yqn(j)+Xdz(j)*Ydn(i)+Xqz(j)*Yqn(i));  
                    end
                end
            end
        end  
    end
    
    Zdp(2:end) = Zdp(1:end-1);
    Zdn(2:end) = Zdn(1:end-1);
    Zdz(2:end) = Zdz(1:end-1);
    Zqp(2:end) = Zqp(1:end-1);
    Zqn(2:end) = Zqn(1:end-1);
    Zqz(2:end) = Zqz(1:end-1);
    
    Zdp(1)     = Zdc(1);
    Zdn(1)     = Zdc(2);
    Zdz(1)     = Zdc(3);
    Zqp(1)     = Zdc(4);
    Zqn(1)     = Zdc(5);
    Zqz(1)     = Zdc(6);
    
    Z_DQN(:,1) = Zdp;
    Z_DQN(:,2) = Zdn;
    Z_DQN(:,3) = Zdz;
    Z_DQN(:,4) = Zqp;
    Z_DQN(:,5) = Zqn;
    Z_DQN(:,6) = Zqz;
    
end

== matlab function DQN_Lib (conflicted copy 2023-11-25 155310)/DQn->ABC19 ==
  data: X_DQN input; th input; abc output; N parameter
%function abc = Mult(Z0,Zdp,Zqp,Zdn,Zqn,Zdz,Zqz,th, N)
function abc = dqn2abc(X_DQN,th,N)

    Xdp = X_DQN(:,1);
    Xdn = X_DQN(:,2);
    Xdz = X_DQN(:,3);
    Xqp = X_DQN(:,4);
    Xqn = X_DQN(:,5);
    Xqz = X_DQN(:,6);

    %Xdc = zeros(1,6);
    Xdc = zeros(6,1);

    Xdc(1) = Xdp(1);
    Xdc(2) = Xdn(1);
    Xdc(3) = Xdz(1);
    Xdc(4) = Xqp(1);
    Xdc(5) = Xqn(1);
    Xdc(6) = Xqz(1);

    Tdqn_a = zeros(3,6);
    
    abc3p = [0;0;0];
    abc3n = [0;0;0];
    abc1p = [0;0;0];
    
    Tda_p = [-0           1     1;
             -sqrt(3/4)  -0.5   1;
              sqrt(3/4)  -0.5   1;];

    Tdqn_a = [Tda_p(:,1)  Tda_p(:,1)  0*Tda_p(:,3)  Tda_p(:,2)  Tda_p(:,2)  2*Tda_p(:,3)]/2;

    abc = Tdqn_a*Xdc;


 
    for i = 1 : N

        Tda_p = [sin(i*th)          cos(i*th);
                 sin(i*th-2*pi/3)   cos(i*th-2*pi/3);
                 sin(i*th+2*pi/3)   cos(i*th+2*pi/3)];
        Tda_n = [sin(-i*th)         cos(-i*th);
                 sin(-i*th-2*pi/3)  cos(-i*th-2*pi/3);
                 sin(-i*th+2*pi/3)  cos(-i*th+2*pi/3)];
        Tda_z = [sin(i*th)          cos(i*th);
                 sin(i*th-0*pi/3)   cos(i*th-0*pi/3);
                 sin(i*th+0*pi/3)   cos(i*th+0*pi/3)];

        abc3p = abc3p + Tda_p*[Xdp(i+1);Xqp(i+1)];
        abc3n = abc3n + Tda_n*[Xdn(i+1);Xqn(i+1)];
        abc1p = abc1p + Tda_z*[Xdz(i+1);Xqz(i+1)];  

    end

    abc = abc+abc3p+abc3n+abc1p;%+abc1n;

== matlab function DQN_Lib (conflicted copy 2023-11-25 155310)/MATLAB Function1 ==
  data: Xdc input size=3; Zdc output size=3; Xdp input; Xdn input; Xdz input; Xqp input; Xqn input; Xqz input; Ydc input size=3; Ydp input; Ydn input; Ydz input; Yqp input; Yqn input; Yqz input; Zdp output; Zdn output; Zdz output; Zqp output; Zqn output; Zqz output; N parameter
function [Zdc,Zdp,Zdn,Zdz,Zqp,Zqn,Zqz]  = SumDQN(Xdc, Xdp, Xdn, Xdz, Xqp, Xqn, Xqz, Ydc, Ydp, Ydn, Ydz, Yqp, Yqn, Yqz, N)
%function [Zdc,Zdp,Zqp,Zdn,Zqn,Zdz,Zqz]  = SumDQN(Xdc, Xdp, Xdn, Xdz, Xqp, Xqn, Xqz, Ydc, Ydp, Ydn, Ydz, Yqp, Yqn, Yqz, N)

    Zdc = zeros(3,1);

    Xdp = [Xdp; zeros(N-numel(Xdp),1)];
    Ydp = [Ydp; zeros(N-numel(Ydp),1)];
    Xqp = [Xqp; zeros(N-numel(Xqp),1)];
    Yqp = [Yqp; zeros(N-numel(Yqp),1)];
      
    Xdn = [Xdn; zeros(N-numel(Xdn),1)];
    Ydn = [Ydn; zeros(N-numel(Ydn),1)];
    Xqn = [Xqn; zeros(N-numel(Xqn),1)];
    Yqn = [Yqn; zeros(N-numel(Yqn),1)];
    
    Xdz = [Xdz; zeros(N-numel(Xdz),1)];
    Ydz = [Ydz; zeros(N-numel(Ydz),1)];
    Xqz = [Xqz; zeros(N-numel(Xqz),1)];
    Yqz = [Yqz; zeros(N-numel(Yqz),1)];
       
    Zdp = zeros(N,1);
    Zdn = zeros(N,1);
    Zqp = zeros(N,1);
    Zqn = zeros(N,1);
    Zdz = zeros(N,1);
    Zqz = zeros(N,1);
   
    Zdc(:) = Xdc(:)+Ydc(:);
   
    for h = 1 : N
        Zdp(h) = Xdp(h)+Ydp(h);
        Zdn(h) = Xdn(h)+Ydn(h);
        Zqp(h) = Xqp(h)+Yqp(h);
        Zqn(h) = Xqn(h)+Yqn(h);
        Zdz(h) = Xdz(h)+Ydz(h);
        Zqz(h) = Xqz(h)+Yqz(h);
    end
end

== matlab function DQN_Lib (conflicted copy 2023-11-25 155310)/DQN Mux1 ==
  data: u input; x output; N parameter
function x = MUX_mat(u, N)

    x = zeros(N+1,6);

    for i = 1 : (N+1)
        x(i,:) = u(6*(i-1)+1:6*(i-1)+6);
    end
    

end

== matlab function DQN_Lib (conflicted copy 2023-11-25 155310)/Der_DQN_Mat ==
  settings: updateMethod=DISCRETE
  data: X_DQN input; Z_DQN output; N parameter; w parameter; EMT parameter; Ts parameter; sw_soft parameter
function Z_DQN   = Der_DQN_Mat(X_DQN, N, w, EMT, Ts, sw_soft)   
    
    persistent Xdp_old;
    persistent Xqp_old;
    persistent Xdn_old;
    persistent Xqn_old;
    persistent Xdz_old;
    persistent Xqz_old;
    persistent firstStep;
    
    Xdp = X_DQN(:,1);
    Xdn = X_DQN(:,2);
    Xdz = X_DQN(:,3);
    Xqp = X_DQN(:,4);
    Xqn = X_DQN(:,5);
    Xqz = X_DQN(:,6);
    
    Z_DQN = zeros(1*N+1,6);
    
    Xdp = [Xdp(2:end); zeros(N-numel(Xdp)+1,1)];
    Xqp = [Xqp(2:end); zeros(N-numel(Xqp)+1,1)];
    Xdn = [Xdn(2:end); zeros(N-numel(Xdn)+1,1)];
    Xqn = [Xqn(2:end); zeros(N-numel(Xqn)+1,1)];
    Xdz = [Xdz(2:end); zeros(N-numel(Xdz)+1,1)];
    Xqz = [Xqz(2:end); zeros(N-numel(Xqz)+1,1)];
       
    dZdp = zeros(N+1,1);
    dZdn = zeros(N+1,1);
    dZqp = zeros(N+1,1);
    dZqn = zeros(N+1,1);
    dZdz = zeros(N+1,1);
    dZqz = zeros(N+1,1);
    
    if(N>0)
        if(isempty(Xdp_old))  Xdp_old     = zeros(N,1); end
        if(isempty(Xqp_old))  Xqp_old     = zeros(N,1); end
        if(isempty(Xdn_old))  Xdn_old     = zeros(N,1); end
        if(isempty(Xqn_old))  Xqn_old     = zeros(N,1); end    
        if(isempty(Xdz_old))  Xdz_old     = zeros(N,1); end
        if(isempty(Xqz_old))  Xqz_old     = zeros(N,1); end    
        if(isempty(firstStep)) firstStep  = 0; end   
    
        for i = 1 : N
            wn = i*w;
            if(EMT)
                if(sw_soft==1 && firstStep == 0)
                Xdp_old(i) = Xdp(i);
                Xqp_old(i) = Xqp(i);
                Xdn_old(i) = Xdn(i);
                Xqn_old(i) = Xqn(i);
                Xdz_old(i) = Xdz(i);
                Xqz_old(i) = Xqz(i);
                else
                dZdp(i) = (Xdp(i)-Xdp_old(i))/Ts;
                Xdp_old(i) = Xdp(i);
                dZqp(i) = (Xqp(i)-Xqp_old(i))/Ts;
                Xqp_old(i) = Xqp(i);
                dZdn(i) = (Xdn(i)-Xdn_old(i))/Ts;
                Xdn_old(i) = Xdn(i);
                dZqn(i) = (Xqn(i)-Xqn_old(i))/Ts;
                Xqn_old(i) = Xqn(i);
                dZdz(i) = (Xdz(i)-Xdz_old(i))/Ts;
                Xdz_old(i) = Xdz(i);
                dZqz(i) = (Xqz(i)-Xqz_old(i))/Ts;
                Xqz_old(i) = Xqz(i);
                end

            end

            dZdp(i) = dZdp(i) + Xqp(i)*(-(wn));
            dZqp(i) = dZqp(i) + Xdp(i)*((wn)); 

            dZdn(i) = dZdn(i) + Xqn(i)*((wn));
            dZqn(i) = dZqn(i) + Xdn(i)*(-(wn)); 

            dZdz(i) = dZdz(i) + Xqz(i)*(-(wn));
            dZqz(i) = dZqz(i) + Xdz(i)*((wn)); 
        end

        firstStep = 1;

        dZdp(2:end) = dZdp(1:end-1);
        dZqp(2:end) = dZqp(1:end-1);
        dZdn(2:end) = dZdn(1:end-1);
        dZqn(2:end) = dZqn(1:end-1);
        dZdz(2:end) = dZdz(1:end-1);
        dZqz(2:end) = dZqz(1:end-1);
    
    end
    dZdp(1)     = 0;
    dZqp(1)     = 0;
    dZdn(1)     = 0;
    dZqn(1)     = 0;
    dZdz(1)     = 0;
    dZqz(1)     = 0;
    
    Z_DQN(:,1) = dZdp;
    Z_DQN(:,2) = dZdn;
    Z_DQN(:,3) = dZdz;
    Z_DQN(:,4) = dZqp;
    Z_DQN(:,5) = dZqn;
    Z_DQN(:,6) = dZqz;

end

== matlab function DQN_Lib (conflicted copy 2023-11-25 155310)/Int_DQN_Mat ==
  settings: updateMethod=DISCRETE
  data: Z_DQN output; X_DQN input; N parameter; dt parameter; w parameter; EMT parameter; InitInt parameter
function Z_DQN   = Int_DQN_Mat(X_DQN, N, dt, w, EMT, InitInt)

    persistent Zdc_old;    
    persistent Xdc_old;   
    persistent Zdp_old;    
    persistent Zqp_old;    
    persistent Zdn_old;    
    persistent Zqn_old;    
    persistent Zdz_old;    
    persistent Zqz_old;  
       
    nrSig  = size(X_DQN,2)/6; 
    Z_DQN = zeros(1*N+1,6*nrSig);


    if(mod(size(X_DQN,2),6) ~= 0)
        error('Invalid input!');
    end
    
    
    for k = 1 : nrSig
    
        ok = (k-1)*6;

        Xdp = X_DQN(:,ok+1);
        Xdn = X_DQN(:,ok+2);
        Xdz = X_DQN(:,ok+3);
        Xqp = X_DQN(:,ok+4);
        Xqn = X_DQN(:,ok+5);
        Xqz = X_DQN(:,ok+6);



        dt2 = dt/2;

        Tad_p2 = (2/3)*[sin(0) sin(0-2*pi/3) sin(0+2*pi/3);  
                       cos(0) cos(0-2*pi/3) cos(0+2*pi/3);];

        Tad_z2 = (1/3)*[sin(0) sin(0) sin(0);  
                       cos(0) cos(0) cos(0);];

        Ta_dqn = [Tad_p2(1,:); Tad_p2(1,:); Tad_z2(1,:); Tad_p2(2,:); Tad_p2(2,:); Tad_z2(2,:)];

        Xdc = zeros(6,1);
        Zdc = zeros(6,1);

        Xdc(1) = Xdp(1);
        Xdc(2) = Xdn(1);
        Xdc(3) = Xdz(1);
        Xdc(4) = Xqp(1);
        Xdc(5) = Xqn(1);
        Xdc(6) = Xqz(1);

        Xdp = [Xdp(2:end); zeros(N-numel(Xdp)+1,1)];
        Xqp = [Xqp(2:end); zeros(N-numel(Xqp)+1,1)];
        Xdn = [Xdn(2:end); zeros(N-numel(Xdn)+1,1)];
        Xqn = [Xqn(2:end); zeros(N-numel(Xqn)+1,1)];
        Xdz = [Xdz(2:end); zeros(N-numel(Xdz)+1,1)];
        Xqz = [Xqz(2:end); zeros(N-numel(Xqz)+1,1)];

        Zdp = zeros(N+1,1);
        Zdn = zeros(N+1,1);
        Zqp = zeros(N+1,1);
        Zqn = zeros(N+1,1);
        Zdz = zeros(N+1,1);
        Zqz = zeros(N+1,1);

        if(isempty(Zdc_old)) 
            
            Zdp_old  = zeros(N,nrSig);% Zdp_old(1) = InitInt(1);
            Zdn_old  = zeros(N,nrSig);% Zdn_old(1) = InitInt(2);
            Zdz_old  = zeros(N,nrSig);% Zdz_old(1) = InitInt(3);
            Zqp_old  = zeros(N,nrSig);% Zqp_old(1) = InitInt(4);
            Zqn_old  = zeros(N,nrSig);% Zqn_old(1) = InitInt(5);
            Zqz_old  = zeros(N,nrSig);% Zqz_old(1) = InitInt(6);
            
            if(isempty(InitInt))
                Zdc_old  = zeros(nrSig*6,1);
            else
                if(nrSig*6 == numel(InitInt))
                    Zdc_old  = InitInt'; 
                else
                    Zdc_old  = zeros(nrSig*6,1);
                end
            end
                        
        end
        if(isempty(Xdc_old)) Xdc_old  = zeros(nrSig*6,1); end

        Zdc(:) = dt2*(Xdc(:)+Xdc_old(ok+1:ok+6))+Zdc_old(ok+1:ok+6);
        Zdc_old(ok+1:ok+6) = Zdc;
        Xdc_old(ok+1:ok+6) = Xdc;


        if(N>0)

            for i = 1 : N
                wn =  i * w; 

                if(EMT)

                    wndt2 = wn*dt2;
                    A = 2/(1+(dt2*wn)^2);

                    %%% POS %%%
                    K1 = dt2*(2*Xdp(i)+Zqp_old(i,k)*wn) + Zdp_old(i,k);
                    K2 = dt2*(2*Xqp(i)-Zdp_old(i,k)*wn) + Zqp_old(i,k);

                    Zdp(i) = A*( K1 + wndt2*K2)/2;
                    Zqp(i) = A*( K2 - wndt2*K1)/2;

                    Zdp_old(i,k) = Zdp(i);
                    Zqp_old(i,k) = Zqp(i); 

                    %%% NEG %%%
                    K1 = dt2*(2*Xdn(i)-Zqn_old(i,k)*wn) + Zdn_old(i,k);
                    K2 = dt2*(2*Xqn(i)+Zdn_old(i,k)*wn) + Zqn_old(i,k);

                    Zdn(i) = A*( K1 - wndt2*K2)/2;
                    Zqn(i) = A*( K2 + wndt2*K1)/2;

                    Zdn_old(i,k) = Zdn(i);
                    Zqn_old(i,k) = Zqn(i);

                    %%% ZERO %%%
                    K1 = dt2*(2*Xdz(i)+Zqz_old(i,k)*wn) + Zdz_old(i,k);
                    K2 = dt2*(2*Xqz(i)-Zdz_old(i,k)*wn) + Zqz_old(i,k);

                    Zdz(i) = A*( K1 + wndt2*K2)/2;
                    Zqz(i) = A*( K2 - wndt2*K1)/2;

                    Zdz_old(i,k) = Zdz(i);
                    Zqz_old(i,k) = Zqz(i);

                else

                    Zdp(i) = (Xqp(i))*(1/(wn));
                    Zqp(i) = (Xdp(i))*(-1/(wn)); 

                    Zdn(i) = (Xqn(i))*(-1/(wn));
                    Zqn(i) = (Xdn(i))*(1/(wn)); 

                    Zdz(i) = (Xqz(i))*(1/(wn));
                    Zqz(i) = (Xdz(i))*(-1/(wn));

                    sT = sin(2*pi/3);
                    cT = cos(2*pi/3);

                    Zdc = Zdc-Ta_dqn*[Zqp(i);-sT*Zdp(i)+cT*Zqp(i);sT*Zdp(i)+cT*Zqp(i)];
                    Zdc = Zdc-Ta_dqn*[Zqn(i);-sT*Zdn(i)+cT*Zqn(i);sT*Zdn(i)+cT*Zqn(i)];
                    Zdc = Zdc-Ta_dqn*[Zqz(i); Zqz(i)             ;Zqz(i)];

                end


            end

            Zdp(2:end) = Zdp(1:end-1);
            Zdn(2:end) = Zdn(1:end-1);
            Zdz(2:end) = Zdz(1:end-1);
            Zqp(2:end) = Zqp(1:end-1);
            Zqn(2:end) = Zqn(1:end-1);
            Zqz(2:end) = Zqz(1:end-1);


        end

        Zdp(1)     = Zdc(1);
        Zdn(1)     = Zdc(2);
        Zdz(1)     = Zdc(3);
        Zqp(1)     = Zdc(4);
        Zqn(1)     = Zdc(5);
        Zqz(1)     = Zdc(6);


        Z_DQN(:,ok+1) = Zdp;
        Z_DQN(:,ok+2) = Zdn;
        Z_DQN(:,ok+3) = Zdz;
        Z_DQN(:,ok+4) = Zqp;
        Z_DQN(:,ok+5) = Zqn;
        Z_DQN(:,ok+6) = Zqz;
    end
end

== matlab function DQN_Lib (conflicted copy 2023-11-25 155310)/Subsystem1/DQN Mux ==
  data: u input; y output; N parameter
function y = MUX_vec(u, N)

    y = zeros((N+1)*6,1);

    for i = 1 : (N+1)*6


        if(i <= 1*(N+1)) %dp
            y(i) = u(mod(i+N,N+1)*6+1);
        elseif(i > 1*(N+1) && i <= 2*(N+1))
            y(i) = u(mod(i+N,N+1)*6+2);
        elseif(i > 2*(N+1) && i <= 3*(N+1))
            y(i) = u(mod(i+N,N+1)*6+3);
        elseif(i > 3*(N+1) && i <= 4*(N+1))
            y(i) = u(mod(i+N,N+1)*6+4);
        elseif(i > 4*(N+1) && i <= 5*(N+1))
            y(i) = u(mod(i+N,N+1)*6+5);
        elseif(i > 5*(N+1) && i <= 6*(N+1))
            y(i) = u(mod(i+N,N+1)*6+6);
        end
    end
    
end

== matlab function DQN_Lib (conflicted copy 2023-11-25 155310)/MATLAB Function2 ==
  settings: updateMethod=DISCRETE
  data: Xdc input; iZdc output; Xdp input; Xdn input; Xdz input; Xqp input; Xqn input; Xqz input; iZdp output; iZdn output; iZdz output; iZqp output; iZqn output; iZqz output; N parameter; w parameter; Ts parameter; IntDC parameter
function [iZdc,iZdp,iZdn,iZdz,iZqp,iZqn,iZqz]  = IntDQN(Xdc, Xdp, Xdn, Xdz, Xqp, Xqn, Xqz, N, w, Ts, IntDC)


    persistent Zdc_old;
    persistent Xdc_old;

    iZdc = zeros(3,1);
    sT = sin(2*pi/3);
    cT = cos(2*pi/3);
    
    Xdp = [Xdp; zeros(N-numel(Xdp),1)];
    Xqp = [Xqp; zeros(N-numel(Xqp),1)];
      
    Xdn = [Xdn; zeros(N-numel(Xdn),1)];
    Xqn = [Xqn; zeros(N-numel(Xqn),1)];
    
    Xdz = [Xdz; zeros(N-numel(Xdz),1)];
    Xqz = [Xqz; zeros(N-numel(Xqz),1)];
       
    iZdp = zeros(N,1);
    iZdn = zeros(N,1);
    iZqp = zeros(N,1);
    iZqn = zeros(N,1);
    iZdz = zeros(N,1);
    iZqz = zeros(N,1);
    
    if(IntDC)


        if(isempty(Zdc_old))  Zdc_old   = zeros(3,1); end
        if(isempty(Xdc_old))  Xdc_old   = zeros(3,1); end

        iZdc(:) = Ts/2*(Xdc(:)+Xdc_old(:))+Zdc_old(:);
        Zdc_old = iZdc;
        Xdc_old = Xdc;
    end
    
    for h = 1 : N
           iZdp(h) = Xqp(h)*(1/(h*w));
           iZqp(h) = Xdp(h)*(-1/(h*w)); 

           
           iZdn(h) = Xqn(h)*(-1/(h*w));
           iZqn(h) = Xdn(h)*(1/(h*w)); 

           
           iZdz(h) = Xqz(h)*(1/(h*w));
           iZqz(h) = Xdz(h)*(-1/(h*w)); 
           if(1)
               iZdc = iZdc-[iZqp(h);-sT*iZdp(h)+cT*iZqp(h);sT*iZdp(h)+cT*iZqp(h)];
               iZdc = iZdc-[iZqn(h);-sT*iZdn(h)+cT*iZqn(h);sT*iZdn(h)+cT*iZqn(h)];
               iZdc = iZdc-[iZqz(h);iZqz(h);iZqz(h)];
           end
    end

    
end

== matlab function DQN_Lib (conflicted copy 2023-11-25 155310)/Gain_DQN_Mat1 ==
  data: X_DQN input; Y_DQN output; R parameter; H parameter; chkInv parameter
function Y_DQN  = Gain_Mat2(X_DQN, R, H, chkInv)
    persistent Rd_DQN;
    persistent Rdc;
    
    Y_DQN = zeros(1*H+1,6);
    ROT = eye(6);
    
    if(~issymmetric(R))
%         row = 0; col = 0;
        [row, col] = find(R);  

        
        if(numel(row) == 1)
            R(col,col) = R(row, col);
            R(row, col) = 0;
            
            d =  0;

            if (row(1) - col(1) == -2 || row(1) - col(1) == 1)
                d = 1;
            elseif(row(1) - col(1) == 2 || row(1) - col(1) == -1)
                d = -1;
            else
                error('Something went wrong!');
            end

            x = sin(d*2*pi/3);

            ROT = ...
            [-0.5,      0,      0,      x,      0,      0;
                0,   -0.5,      0,      0,      x,      0;
                0,      0,      1,      0,      0,      0;
               -x,      0,      0,   -0.5,      0,      0;
                0,     -x,      0,      0,   -0.5,      0;
                0,      0,      0,      0,      0,      1];
        
        end

    end
    

    
    if(isempty(Rd_DQN))
        Rd = diag(diag(R));
        Rm = R - Rd;
        Tad_p = [0      -sqrt(1/3)   sqrt(1/3);
                (2/3)   -(1/3)      -(1/3);
                (1/3)    (1/3)       (1/3)];

        Tda_p = [-0           1     1;
                 -sqrt(3/4)  -0.5   1;
                  sqrt(3/4)  -0.5   1;];
              
        Rdq = Tad_p*Rd*Tda_p;
        Rm_dq = Tad_p*Rm*Tda_p;
        Rm_DQN = -eye(6)*Rm_dq(3,3)/2;
        Rm_DQN(3,3) = Rm_dq(3,3);
        Rm_DQN(6,6) = Rm_dq(3,3);
        
        Rd_DQN = [ Rdq(3,3)	-Rdq(3,2)	 Rdq(3,2)	 0          -Rdq(3,1)	 Rdq(3,1);
                -Rdq(3,2)	 Rdq(3,3)	-Rdq(3,2)	-Rdq(3,1)	 0           Rdq(3,1);
                 Rdq(3,2)	-Rdq(3,2)	 Rdq(3,3)	-Rdq(3,1)	 Rdq(3,1)	 0;
                 0          -Rdq(3,1)	-Rdq(3,1)	 Rdq(3,3)	 Rdq(3,2)	 Rdq(3,2);
                -Rdq(3,1)	 0           Rdq(3,1)	 Rdq(3,2)	 Rdq(3,3)	 Rdq(3,2);
                 Rdq(3,1)	 Rdq(3,1)	 0           Rdq(3,2)	 Rdq(3,2)	 Rdq(3,3);];
             
        Rd_DQN = Rd_DQN + Rm_DQN;
             
        Tdqn_a = [Tda_p(:,1)  Tda_p(:,1)  0*Tda_p(:,3)  Tda_p(:,2)  Tda_p(:,2)  2*Tda_p(:,3)]/2;
        Ta_dqn = [Tad_p(1,:); Tad_p(1,:); 0*Tad_p(3,:); Tad_p(2,:); Tad_p(2,:); Tad_p(3,:)];
        
        if(chkInv)
            Rd_DQN = eye(6)/Rd_DQN;
            Rdc = (Ta_dqn*(eye(3)/R)*Tdqn_a);
        else
            Rdc = (Ta_dqn*R*Tdqn_a);
        end
    end

    Y_DQN(1,:)     = (Rdc*X_DQN(1,:)')';
    if(H>0)
        Y_DQN(2:end,:) = (Rd_DQN*X_DQN(2:end,:)')'*ROT;
    end
end


% function Y  = Gain(X, A, H)
% 
%     Y = zeros(3+6*H,1);
% 
%     for i = 1 : H
%         
%         Y(4 + (i-1)*6) = X(3+i+0*H);
%         Y(5 + (i-1)*6) = X(3+i+1*H);
%         Y(6 + (i-1)*6) = X(3+i+2*H);
%         Y(7 + (i-1)*6) = X(3+i+3*H);
%         Y(8 + (i-1)*6) = X(3+i+4*H);
%         Y(9 + (i-1)*6) = X(3+i+5*H);
% 
%         Y(4+6*(i-1):4+(i)*6-1) = A(4:end, 4:end)*Y(4+6*(i-1):4+(i)*6-1);
%         
%         X(3+i+0*H) = Y(4 + (i-1)*6);
%         X(3+i+1*H) = Y(5 + (i-1)*6);
%         X(3+i+2*H) = Y(6 + (i-1)*6);
%         X(3+i+3*H) = Y(7 + (i-1)*6);
%         X(3+i+4*H) = Y(8 + (i-1)*6);
%         X(3+i+5*H) = Y(9 + (i-1)*6);
%     end
%     
% 
% 
%     Y(1:3) = A(1:3,1:3) * X(1:3);
% 
%     Y(4:end) = X(4:end);
%     
% end
